simulink subsystem "euler"  (R2024b)
settings: Solver=VariableStepAuto  StartTime=0.0  StopTime=10.0  RelTol=1e-3
undefined symbols (not defined in the file): DiscIntNeverNeededParam
settings Model: Creator=yagiz  LastModifiedBy=yagiz

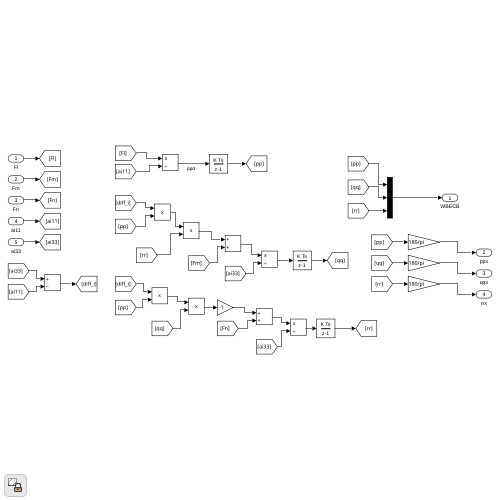
[thumbnail: Simulink's stored preview of the top-level diagram]
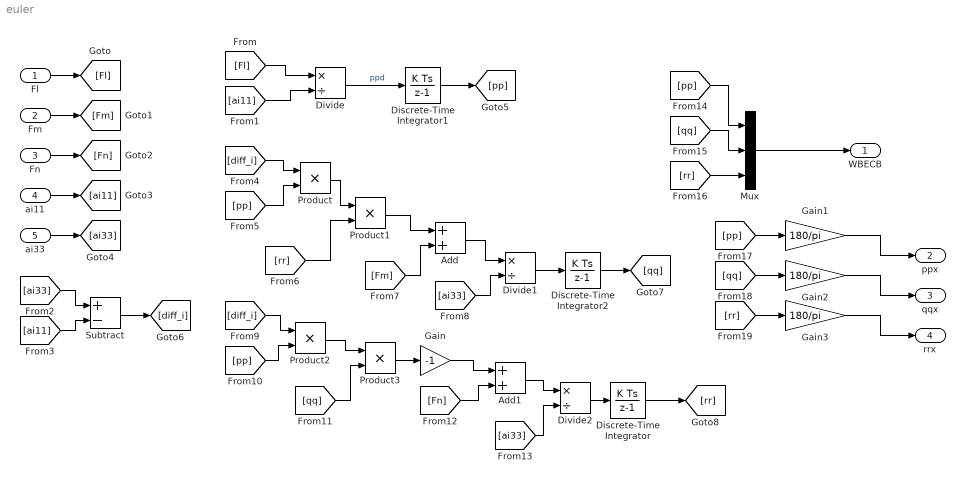
== system euler ==
  Fl : Inport
  Fm : Inport  Port=2
  Fn : Inport  Port=3
  ai11 : Inport  Port=4
  ai33 : Inport  Port=5
  Add : Sum
  Add1 : Sum
  Discrete-Time Integrator : DiscreteIntegrator  SampleTime=0.001  ICPrevOutput=DiscIntNeverNeededParam  ICPrevScaledInput=DiscIntNeverNeededParam
  Discrete-Time Integrator1 : DiscreteIntegrator  SampleTime=0.001  ICPrevOutput=DiscIntNeverNeededParam  ICPrevScaledInput=DiscIntNeverNeededParam
  Discrete-Time Integrator2 : DiscreteIntegrator  SampleTime=0.001  ICPrevOutput=DiscIntNeverNeededParam  ICPrevScaledInput=DiscIntNeverNeededParam
  Divide : Product  Inputs=*/
  Divide1 : Product  Inputs=*/
  Divide2 : Product  Inputs=*/
  Gain : Gain  Gain=-1
  Gain1 : Gain  Gain=180/pi
  Gain2 : Gain  Gain=180/pi
  Gain3 : Gain  Gain=180/pi
  Mux : Mux  Inputs=3
  Product{,1..3} (4 alike) : Product
  Subtract : Sum  Inputs=+-
  WBECB : Outport
  ppx : Outport  Port=2
  qqx : Outport  Port=3
  rrx : Outport  Port=4
  wires:
  Fl/1 -> [Fl]
  Fm/1 -> [Fm]
  Fn/1 -> [Fn]
  ai11/1 -> [ai11]
  ai33/1 -> [ai33]
  [Fl] -> Divide/1
  [ai11] -> Divide/2
  Divide/1 -> Discrete-Time Integrator1/1  "ppd"
  Discrete-Time Integrator1/1 -> [pp]
  [ai33] -> Subtract/1
  [ai11] -> Subtract/2
  Subtract/1 -> [diff_i]
  [diff_i] -> Product/1
  [pp] -> Product/2
  Product/1 -> Product1/1
  [rr] -> Product1/2
  Product1/1 -> Add/1
  [Fm] -> Add/2
  Add/1 -> Divide1/1
  [ai33] -> Divide1/2
  Divide1/1 -> Discrete-Time Integrator2/1
  Discrete-Time Integrator2/1 -> [qq]
  [diff_i] -> Product2/1
  [pp] -> Product2/2
  Product2/1 -> Product3/1
  [qq] -> Product3/2
  Product3/1 -> Gain/1
  Gain/1 -> Add1/1
  [Fn] -> Add1/2
  Add1/1 -> Divide2/1
  [ai33] -> Divide2/2
  Divide2/1 -> Discrete-Time Integrator/1
  Discrete-Time Integrator/1 -> [rr]
  [pp] -> Mux/1
  [qq] -> Mux/2
  [rr] -> Mux/3
  Mux/1 -> WBECB/1
  [pp] -> Gain1/1
  Gain1/1 -> ppx/1
  [qq] -> Gain2/1
  Gain2/1 -> qqx/1
  Gain3/1 -> rrx/1
  [rr] -> Gain3/1
